simulink model "RobotArm"  (R2022b)
settings: Solver=FixedStepAuto  StartTime=0.0  StopTime=20  FixedStep=0.01  RelTol=1e-3
settings Model: Creator=Admins  LastModifiedBy=Admins
settings DataIOCC: ReturnWorkspaceOutputs=off

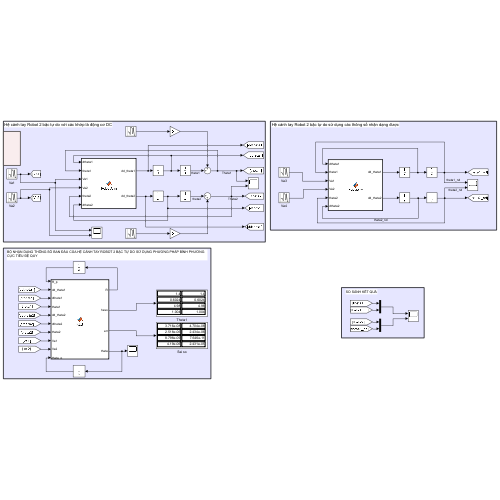
[thumbnail: Simulink's stored preview of the top-level diagram]
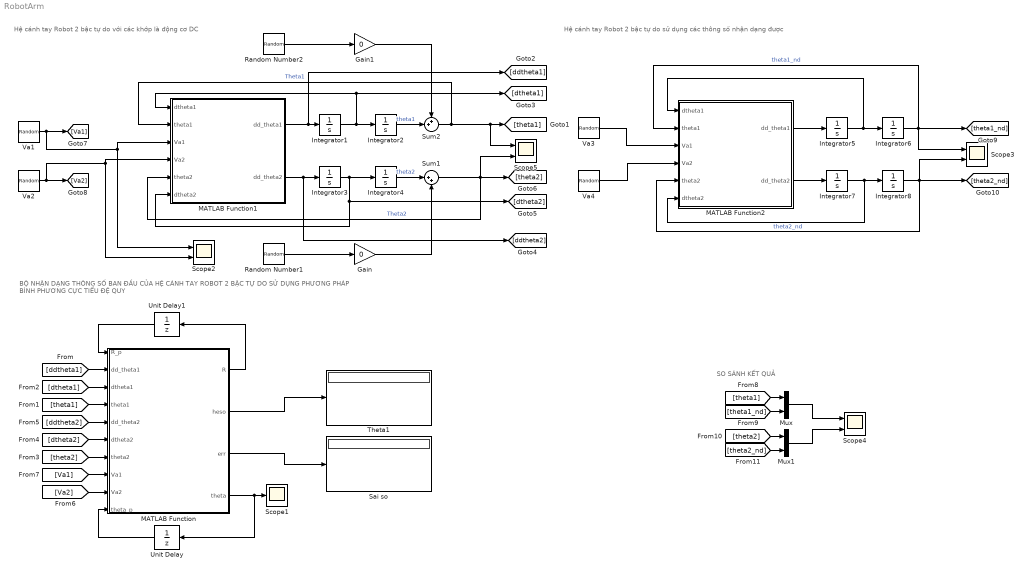
== system RobotArm ==
  note: SO SÁNH KẾT QUẢ
  note: BỘ NHẬN DẠNG THÔNG SỐ BAN ĐẦU CỦA HỆ CÁNH TAY ROBOT 2 BẬC TỰ DO SỬ DỤNG PHƯƠNG PHÁP BÌNH PHƯƠNG CỰC TIỂU ĐỆ QUY
  note: Hệ cánh tay Robot 2 bậc tự do với các khớp là động cơ DC
  note: Hệ cánh tay Robot 2 bậc tự do sử dụng các thông số nhận dạng được
  Gain : Gain  Gain=0
  Gain1 : Gain  Gain=0
  Integrator{1,3,5,7} (4 alike) : Integrator
  Integrator{2,4,6,8} (4 alike) : Integrator  InitialCondition=pi/4  UpperSaturationLimit=pi/2  LowerSaturationLimit=-pi/2
  MATLAB Function : MATLAB Function  TreatAsAtomicUnit=on
  MATLAB Function1 : MATLAB Function  TreatAsAtomicUnit=on
  MATLAB Function2 : MATLAB Function  TreatAsAtomicUnit=on
  Mux : Mux  Inputs=2
  Mux1 : Mux  Inputs=2
  Random Number1 : RandomNumber  Variance=0.01  SampleTime=0.01
  Random Number2 : RandomNumber  Variance=0.01  SampleTime=0.01
  Sai so : Display
  Scope1 : Scope
  Scope{2..5} (4 alike) : Scope  NumInputPorts=2
  Sum1 : Sum  Inputs=|++
  Sum2 : Sum  Inputs=++|
  Theta1 : Display
  Unit Delay : UnitDelay  InitialCondition=zeros(11,1)  SampleTime=-1  HasFrameUpgradeWarning=on
  Unit Delay1 : UnitDelay  InitialCondition=diag([1,1,1,1,1,1,1,1,1,1,1])*10  SampleTime=-1  HasFrameUpgradeWarning=on
  Va{1..4} (4 alike) : RandomNumber  Variance=6.8  SampleTime=0.01
  wires:
  Integrator1/1 -> MATLAB Function1/1(dtheta1), [dtheta1], Integrator2/1
  MATLAB Function1/1(dd_theta1) -> [ddtheta1], Integrator1/1
  Integrator2/1 -> Sum2/2  "theta1"
  Integrator3/1 -> Integrator4/1, MATLAB Function1/6(dtheta2), [dtheta2]
  MATLAB Function1/2(dd_theta2) -> [ddtheta2], Integrator3/1
  Integrator4/1 -> Sum1/1  "theta2"
  MATLAB Function/4(theta) -> Unit Delay/1, Scope1/1
  MATLAB Function/1(R) -> Unit Delay1/1
  Unit Delay/1 -> MATLAB Function/10(theta_p)
  Unit Delay1/1 -> MATLAB Function/1(R_p)
  [ddtheta1] -> MATLAB Function/2(dd_theta1)
  [theta1] -> MATLAB Function/4(theta1)
  [dtheta1] -> MATLAB Function/3(dtheta1)
  [theta2] -> MATLAB Function/7(theta2)
  [dtheta2] -> MATLAB Function/6(dtheta2)
  [ddtheta2] -> MATLAB Function/5(dd_theta2)
  [Va1] -> MATLAB Function/8(Va1)
  [Va2] -> MATLAB Function/9(Va2)
  MATLAB Function/2(heso) -> Theta1/1
  Va1/1 -> [Va1], Scope2/1, MATLAB Function1/3(Va1)
  Va2/1 -> Scope2/2, MATLAB Function1/4(Va2), [Va2]
  Va4/1 -> MATLAB Function2/4(Va2)
  Integrator7/1 -> Integrator8/1, MATLAB Function2/6(dtheta2)
  Integrator6/1 -> MATLAB Function2/2(theta1), [theta1_nd], Scope3/1  "theta1_nd"
  MATLAB Function2/2(dd_theta2) -> Integrator7/1
  Integrator8/1 -> [theta2_nd], Scope3/2, MATLAB Function2/5(theta2)  "theta2_nd"
  MATLAB Function2/1(dd_theta1) -> Integrator5/1
  Va3/1 -> MATLAB Function2/3(Va1)
  Integrator5/1 -> MATLAB Function2/1(dtheta1), Integrator6/1
  Mux/1 -> Scope4/1
  Mux1/1 -> Scope4/2
  [theta1] -> Mux/1
  [theta1_nd] -> Mux/2
  [theta2] -> Mux1/1
  [theta2_nd] -> Mux1/2
  Random Number1/1 -> Gain/1
  Sum1/1 -> Scope5/2, MATLAB Function1/5(theta2), [theta2]  "Theta2"
  Sum2/1 -> Scope5/1, [theta1], MATLAB Function1/2(theta1)  "Theta1"
  Random Number2/1 -> Gain1/1
  Gain/1 -> Sum1/2
  Gain1/1 -> Sum2/1
  MATLAB Function/3(err) -> Sai so/1

== matlab function RobotArm/MATLAB Function1 ==
  data: dtheta1 input; theta1 input; Va1 input; Va2 input; theta2 input; dtheta2 input; dd_theta1 output; dd_theta2 output
function [dd_theta1, dd_theta2]   = RobotArm( dtheta1, theta1,  Va1, Va2, theta2, dtheta2)
m1 = 0.6;
m2 = 0.6
L1 = 1.4;
L2 = 1.4;

I1 = 1;
I2 = 1;  

kt1 = 0.02;
kt2 = 0.02;

kb1 = 0.02;
kb2 = 0.02;

B1 = 4;
B2 = 2;
Ra1 = 5;
Ra2 = 5;


g = 9.8;



M = [m1*L1^2 + m2*(L1^2 + 2*L1*L2*cos(theta2) + L2^2) + I1,     m2*(L1*L2*cos(theta2) + L2^2);...
     m2*(L1*L2*cos(theta2) + L2^2)                        ,     m2*L2^2 + I2                  ];
 
V = [-m2*L1*L2*sin(theta2)*(2*dtheta1*dtheta2 + dtheta2^2) + (kt1*kb1/Ra1 + B1)*dtheta1;
               m2*L1*L2*sin(theta2)*dtheta1^2 + (kt2*kb2/Ra2 + B2)*dtheta2             ];

G = [(m1 + m2)*L1*g*cos(theta1) + m2*g*L2*cos(theta1 + theta2) ;
                  m2*g*L2*cos(theta1 + theta2)                ];

A = [ kt1/Ra1,     0     ;
         0   ,  kt2/Ra2 ];
Va = [Va1;
      Va2];

dd_theta = inv(M)*(A*Va - V - G);
dd_theta1 = dd_theta(1);
dd_theta2 = dd_theta(2);

end

== matlab function RobotArm/MATLAB Function ==
  data: R_p input; R output; heso output; err output; dd_theta1 input; dtheta1 input; theta1 input; dd_theta2 input; dtheta2 input; theta2 input; Va1 input; Va2 input; theta_p input; theta output
function [R, heso, err, theta] = RLS(R_p,dd_theta1, dtheta1, theta1, dd_theta2, dtheta2, theta2, Va1, Va2, theta_p)
lamda=0.98;
g = 9.8;
kt1 = 0.02;
kt2 = 0.02;
kb1 = 0.02;
kb2 = 0.02;
B1 = 4;
B2 = 2;

Va = [Va1;
      Va2];
y = Va; 

phi = [dd_theta1,  (dd_theta1 + dd_theta2), (2*cos(theta2)*dd_theta1 + cos(theta2)*dd_theta2 - sin(theta2)*(2*dtheta1*dtheta2 + dtheta2^2)), cos(theta1), cos(theta1 + theta2),  dtheta1,      0,               0,                                  0,                                 0,              0    ;
       0,                    0,                                    0,                                                                            0,                 0,               0  , dd_theta2, (dd_theta1 + dd_theta2), cos(theta2)*dd_theta1 + dtheta1^2*sin(theta2), cos(theta1 + theta2), dtheta2  ];

%teta = [m1*L1^2 + m2*L1^2 + I1;
%         m2*L2^2;
%         m2*L1*L2;
%         (m1 + m2)*L1*g;
%         m2*g*L2;
%         (kt1*kb1/Ra1 + B1);
%         
%          I2
%         m2*L2^2;
%         m2*L1*L2;
%         cos(theta1 + theta2)
%         (kt2*kb2/Ra2 + B2)

esi1 = y - phi * theta_p;
theta = (theta_p + (inv(R_p)*phi'*esi1));
R = lamda*R_p  + phi'*phi;

L2 = theta(2)/theta(5)*g;
L1 = theta(3)/theta(5)*g;
Ra1 = theta(6)*(kt1/B1) - kb1;
Ra2 = theta(11)*(kt2/B2) - kb2;
m2 = theta(2)*(kt1/Ra1)/L2^2;
m1 = theta(4)*(kt1/Ra1)/(L1*g) - m2;
I1 = theta(1)*(kt1/Ra1) - (m1*L1^2 + m2*L1^2);
I2 = theta(7)*kt2/Ra2;

heso_chuan = [1.4000,    1.4000;
              0.6024,    0.6024;
              4.9801,    4.9802;
              1.0040,    1.0040];

heso = [ L1, L2 ;
          m1, m2 ;
          Ra1, Ra2;
          I1, I2 ]

err = abs((heso_chuan-heso))

if sum(abs(err),"all") > 0.02
    [X, ind] = max(abs(err), [], 'all', 'linear');
    index = ind
    heso_ = { 'L1', 'L2' ;'m1', 'm2' ;'Ra1', 'Ra2';'I1', 'I2'};
    thongso_batthuong = heso_{index}

end

end

== matlab function RobotArm/MATLAB Function2 ==
  data: dtheta1 input; theta1 input; Va1 input; Va2 input; theta2 input; dtheta2 input; dd_theta1 output; dd_theta2 output
function [dd_theta1, dd_theta2]   = RobotArm( dtheta1, theta1,  Va1, Va2, theta2, dtheta2)

heso =  [1.4000,    1.4000;
          0.6024,    0.6024;
          4.9801,    4.9802;
          1.0040,    1.0040];

L1 = heso(1,1);
L2 = heso(1,2);
m1 = heso(2,1);
m2 = heso(2,2);
Ra1 = heso(3,1);
Ra2 = heso(3,2);
I1 = heso(4,1);
I2 = heso(4,2);

% heso = [ L1, L2 ;
%           m1, m2 ;
%           Ra1, Ra2;
%           I1, I2 ]

kt1 = 0.02;
kt2 = 0.02;
kb1 = 0.02;
kb2 = 0.02;
B1 = 4;
B2 = 2;
g = 9.8;

M = [m1*L1^2 + m2*(L1^2 + 2*L1*L2*cos(theta2) + L2^2) + I1,     m2*(L1*L2*cos(theta2) + L2^2);...
     m2*(L1*L2*cos(theta2) + L2^2)                        ,     m2*L2^2 + I2                  ];
V = [-m2*L1*L2*sin(theta2)*(2*dtheta1*dtheta2 + dtheta2^2) + (kt1*kb1/Ra1 + B1)*dtheta1;
               m2*L1*L2*sin(theta2)*dtheta1^2 + (kt2*kb2/Ra2 + B2)*dtheta2             ];
G = [(m1 + m2)*L1*g*cos(theta1) + m2*g*L2*cos(theta1 + theta2) ;
                  m2*g*L2*cos(theta1 + theta2)                ];
A = [ kt1/Ra1,     0     ;
         0   ,  kt2/Ra2 ];
Va = [Va1;
      Va2];

dd_theta = inv(M)*(A*Va - V - G);
dd_theta1 = dd_theta(1);
dd_theta2 = dd_theta(2);

end
